simulink model "Simulink_TEP"  (R2024a)
settings: Solver=FixedStepAuto  StartTime=0.0  StopTime=5  FixedStep=1/3600  RelTol=1e-3
model workspace (MAT data in the model file):
  AD : Simulink.Parameter (value not decoded)
  AG : Simulink.Parameter (value not decoded)
  AH : Simulink.Parameter (value not decoded)
  AV : Simulink.Parameter (value not decoded)
  AVP : Simulink.Parameter (value not decoded)
  BCHL : Simulink.Parameter (value not decoded)
  BCHV : Simulink.Parameter (value not decoded)
  BD : Simulink.Parameter (value not decoded)
  BG : Simulink.Parameter (value not decoded)
  BH : Simulink.Parameter (value not decoded)
  BVP : Simulink.Parameter (value not decoded)
  CD : Simulink.Parameter (value not decoded)
  CG : Simulink.Parameter (value not decoded)
  CH : Simulink.Parameter (value not decoded)
  CVP : Simulink.Parameter (value not decoded)
  XMW : Simulink.Parameter (value not decoded)
symbols that are objects in the model workspace (value not decoded): AD, AG, AH, AV, AVP, BD, BG, BH, BVP, CD, CG, CH, CVP, XMW
undefined symbols (not defined in the file or in its folder): magnitude, SETPT, XMEAS, XMV
libraries: mylib x165, dspindex x17
(part 7 of 10)

== system Simulink_TEP/Subsystem/Braatz/ 7 ==
  XMEAS : Inport
  Bus Selector : BusSelector  OutputSignals=signal4.XMEAS(17)
  CONTROL 11 : Subsystem
  XMV(11) : Outport  VectorParamsAs1DForOutWhenUnconnected=off
  wires:
  CONTROL 11/1(XMV(11)) -> XMV(11)/1
  XMEAS/1 -> Bus Selector/1
  Bus Selector/1 -> CONTROL 11/1(XMEAS(17))  "<XMEAS(17)>"

== system Simulink_TEP/Subsystem/Braatz/ 8 ==
  XMEAS : Inport
  Bus Selector : BusSelector  OutputSignals=XMEAS(21),signal2.XMEAS(9)
  CONTROL 10 : Subsystem
  CONTROL 18 : Subsystem
  XMV(10) : Outport  VectorParamsAs1DForOutWhenUnconnected=off
  wires:
  CONTROL 10/1(XMV(10)) -> XMV(10)/1
  CONTROL 18/1(SETPT(10)) -> CONTROL 10/2(SETPT(10))
  XMEAS/1 -> Bus Selector/1
  Bus Selector/1 -> CONTROL 10/1(XMEAS(21))  "<XMEAS(21)>"
  Bus Selector/2 -> CONTROL 18/1(XMEAS(9))  "<XMEAS(9)>"

== system Simulink_TEP/Subsystem/Braatz/ 9 ==
  XMEAS : Inport
  Bus Selector : BusSelector  OutputSignals=signal4.XMEAS(19),signal4.XMEAS(18),signal10.XMEAS(38)
  CONTROL 16 : Subsystem
  CONTROL 20 : Subsystem
  CONTROL 9 : Subsystem
  XMV(9) : Outport  VectorParamsAs1DForOutWhenUnconnected=off
  wires:
  CONTROL 9/1(XMV(9)) -> XMV(9)/1
  CONTROL 16/1(SETPT(9)) -> CONTROL 9/2(SETPT(9))
  XMEAS/1 -> Bus Selector/1
  Bus Selector/1 -> CONTROL 9/1(XMEAS(19))  "<XMEAS(19)>"
  Bus Selector/2 -> CONTROL 16/1(XMEAS(18))  "<XMEAS(18)>"
  Bus Selector/3 -> CONTROL 20/1(XMEAS(38))  "<XMEAS(38)>"
  CONTROL 20/1(SETPT(16)) -> CONTROL 16/2(SETPT(16))

== system Simulink_TEP/Disturbances/Subsystem1/Subsystem2/If Action Subsystem ==
  IDWLK : Inport
  "DIST " : Inport  Port=2
  TESUB7 : Inport  Port=3
  Action Port : ActionPort  ActionPortLabel=elseif(u1 >= u2)
  Bus Creator : BusCreator  Inputs=6
  Bus Selector : BusSelector  OutputSignals=ADIST,BDIST,CDIST,DDIST,TNEXT,TLAST
  Disturbance parameters I=1-9 : mylib/Disturbance parameters I=1-9  SystemSampleTime=-1  VariantActivationTime=update diagram  AllowFlexibleInterface=on  Latency=0  AutoFrameSizeCalculation=off
  Subsystem : Subsystem
      mask Display: color('Blue'),disp('Disturbance constants')
  DIST_NEW : Outport  PortDimensions=6  VectorParamsAs1DForOutWhenUnconnected=off
  wires:
  Disturbance parameters I=1-9/5 -> Bus Creator/5  "TNEXT"
  Bus Creator/1 -> DIST_NEW/1
  IDWLK/1 -> Disturbance parameters I=1-9/7
  Bus Selector/1 -> Disturbance parameters I=1-9/1  "<ADIST>"
  Subsystem/1(Out1) -> Disturbance parameters I=1-9/8
  Bus Selector/2 -> Disturbance parameters I=1-9/2  "<BDIST>"
  Disturbance parameters I=1-9/1 -> Bus Creator/1  "ADIST"
  Bus Selector/6 -> Disturbance parameters I=1-9/6  "<TLAST>"
  Bus Selector/5 -> Disturbance parameters I=1-9/5  "<TNEXT>"
  Disturbance parameters I=1-9/4 -> Bus Creator/4  "DDIST"
  Disturbance parameters I=1-9/3 -> Bus Creator/3  "CDIST"
  Bus Selector/4 -> Disturbance parameters I=1-9/4  "<DDIST>"
  Disturbance parameters I=1-9/6 -> Bus Creator/6  "TLAST"
  Bus Selector/3 -> Disturbance parameters I=1-9/3  "<CDIST>"
  "DIST "/1 -> Bus Selector/1
  Disturbance parameters I=1-9/2 -> Bus Creator/2  "BDIST"
  TESUB7/1 -> Disturbance parameters I=1-9/9

== system Simulink_TEP/Disturbances/Subsystem1/Subsystem2/If Action Subsystem1 ==
  Action Port : ActionPort  ActionPortLabel=if(u1 == 0)
  Subsystem1 : Subsystem
  DIST : Outport  VectorParamsAs1DForOutWhenUnconnected=off
  wires:
  Subsystem1/1(DIST) -> DIST/1

== system Simulink_TEP/Disturbances/Subsystem10/Subsystem3/If Action Subsystem ==
  IDWLK : Inport
  "DIST " : Inport  Port=2
  TESUB7 : Inport  Port=3
  Action Port : ActionPort  ActionPortLabel=elseif(u1 >= u2)
  Bus Creator : BusCreator  Inputs=6
  Bus Selector : BusSelector  OutputSignals=ADIST,BDIST,CDIST,DDIST,TNEXT,TLAST
  Disturbance parameters I=10-12 : mylib/Disturbance parameters I=10-12  SystemSampleTime=-1  VariantActivationTime=update diagram  AllowFlexibleInterface=on  Latency=0  AutoFrameSizeCalculation=off
  Subsystem2 : Subsystem
      mask Display: color('Blue'),disp('Disturbance constants')
  DIST_NEW : Outport  PortDimensions=6  VectorParamsAs1DForOutWhenUnconnected=off
  SWLK : Outport  Port=2  VectorParamsAs1DForOutWhenUnconnected=off
  wires:
  Disturbance parameters I=10-12/5 -> Bus Creator/5  "TNEXT"
  Bus Creator/1 -> DIST_NEW/1
  IDWLK/1 -> Disturbance parameters I=10-12/7
  Bus Selector/1 -> Disturbance parameters I=10-12/1  "<ADIST>"
  Subsystem2/1(Out1) -> Disturbance parameters I=10-12/8
  Bus Selector/2 -> Disturbance parameters I=10-12/2  "<BDIST>"
  Disturbance parameters I=10-12/1 -> Bus Creator/1  "ADIST"
  Bus Selector/6 -> Disturbance parameters I=10-12/6  "<TLAST>"
  Bus Selector/5 -> Disturbance parameters I=10-12/5  "<TNEXT>"
  Disturbance parameters I=10-12/4 -> Bus Creator/4  "DDIST"
  Disturbance parameters I=10-12/3 -> Bus Creator/3  "CDIST"
  Bus Selector/4 -> Disturbance parameters I=10-12/4  "<DDIST>"
  Disturbance parameters I=10-12/6 -> Bus Creator/6  "TLAST"
  Bus Selector/3 -> Disturbance parameters I=10-12/3  "<CDIST>"
  "DIST "/1 -> Bus Selector/1
  Disturbance parameters I=10-12/2 -> Bus Creator/2  "BDIST"
  TESUB7/1 -> Disturbance parameters I=10-12/9
  Disturbance parameters I=10-12/7 -> SWLK/1  "SWLK"

== system Simulink_TEP/Disturbances/Subsystem10/Subsystem3/If Action Subsystem1 ==
  Action Port : ActionPort  ActionPortLabel=if(u1 == 0)
  Subsystem1 : Subsystem
  DIST : Outport  VectorParamsAs1DForOutWhenUnconnected=off
  wires:
  Subsystem1/1(DIST) -> DIST/1

== system Simulink_TEP/Disturbances/Subsystem11/Subsystem3/If Action Subsystem ==
  IDWLK : Inport
  "DIST " : Inport  Port=2
  TESUB7 : Inport  Port=3
  Action Port : ActionPort  ActionPortLabel=elseif(u1 >= u2)
  Bus Creator : BusCreator  Inputs=6
  Bus Selector : BusSelector  OutputSignals=ADIST,BDIST,CDIST,DDIST,TNEXT,TLAST
  Disturbance parameters I=10-12 : mylib/Disturbance parameters I=10-12  SystemSampleTime=-1  VariantActivationTime=update diagram  AllowFlexibleInterface=on  Latency=0  AutoFrameSizeCalculation=off
  Subsystem2 : Subsystem
      mask Display: color('Blue'),disp('Disturbance constants')
  DIST_NEW : Outport  PortDimensions=6  VectorParamsAs1DForOutWhenUnconnected=off
  SWLK : Outport  Port=2  VectorParamsAs1DForOutWhenUnconnected=off
  wires:
  Disturbance parameters I=10-12/5 -> Bus Creator/5  "TNEXT"
  Bus Creator/1 -> DIST_NEW/1
  IDWLK/1 -> Disturbance parameters I=10-12/7
  Bus Selector/1 -> Disturbance parameters I=10-12/1  "<ADIST>"
  Subsystem2/1(Out1) -> Disturbance parameters I=10-12/8
  Bus Selector/2 -> Disturbance parameters I=10-12/2  "<BDIST>"
  Disturbance parameters I=10-12/1 -> Bus Creator/1  "ADIST"
  Bus Selector/6 -> Disturbance parameters I=10-12/6  "<TLAST>"
  Bus Selector/5 -> Disturbance parameters I=10-12/5  "<TNEXT>"
  Disturbance parameters I=10-12/4 -> Bus Creator/4  "DDIST"
  Disturbance parameters I=10-12/3 -> Bus Creator/3  "CDIST"
  Bus Selector/4 -> Disturbance parameters I=10-12/4  "<DDIST>"
  Disturbance parameters I=10-12/6 -> Bus Creator/6  "TLAST"
  Bus Selector/3 -> Disturbance parameters I=10-12/3  "<CDIST>"
  "DIST "/1 -> Bus Selector/1
  Disturbance parameters I=10-12/2 -> Bus Creator/2  "BDIST"
  TESUB7/1 -> Disturbance parameters I=10-12/9
  Disturbance parameters I=10-12/7 -> SWLK/1  "SWLK"

== system Simulink_TEP/Disturbances/Subsystem11/Subsystem3/If Action Subsystem1 ==
  Action Port : ActionPort  ActionPortLabel=if(u1 == 0)
  Subsystem1 : Subsystem
  DIST : Outport  VectorParamsAs1DForOutWhenUnconnected=off
  wires:
  Subsystem1/1(DIST) -> DIST/1

== system Simulink_TEP/Disturbances/Subsystem12/Subsystem3/If Action Subsystem ==
  IDWLK : Inport
  "DIST " : Inport  Port=2
  TESUB7 : Inport  Port=3
  Action Port : ActionPort  ActionPortLabel=elseif(u1 >= u2)
  Bus Creator : BusCreator  Inputs=6
  Bus Selector : BusSelector  OutputSignals=ADIST,BDIST,CDIST,DDIST,TNEXT,TLAST
  Disturbance parameters I=10-12 : mylib/Disturbance parameters I=10-12  SystemSampleTime=-1  VariantActivationTime=update diagram  AllowFlexibleInterface=on  Latency=0  AutoFrameSizeCalculation=off
  Subsystem2 : Subsystem
      mask Display: color('Blue'),disp('Disturbance constants')
  DIST_NEW : Outport  PortDimensions=6  VectorParamsAs1DForOutWhenUnconnected=off
  SWLK : Outport  Port=2  VectorParamsAs1DForOutWhenUnconnected=off
  wires:
  Disturbance parameters I=10-12/5 -> Bus Creator/5  "TNEXT"
  Bus Creator/1 -> DIST_NEW/1
  IDWLK/1 -> Disturbance parameters I=10-12/7
  Bus Selector/1 -> Disturbance parameters I=10-12/1  "<ADIST>"
  Subsystem2/1(Out1) -> Disturbance parameters I=10-12/8
  Bus Selector/2 -> Disturbance parameters I=10-12/2  "<BDIST>"
  Disturbance parameters I=10-12/1 -> Bus Creator/1  "ADIST"
  Bus Selector/6 -> Disturbance parameters I=10-12/6  "<TLAST>"
  Bus Selector/5 -> Disturbance parameters I=10-12/5  "<TNEXT>"
  Disturbance parameters I=10-12/4 -> Bus Creator/4  "DDIST"
  Disturbance parameters I=10-12/3 -> Bus Creator/3  "CDIST"
  Bus Selector/4 -> Disturbance parameters I=10-12/4  "<DDIST>"
  Disturbance parameters I=10-12/6 -> Bus Creator/6  "TLAST"
  Bus Selector/3 -> Disturbance parameters I=10-12/3  "<CDIST>"
  "DIST "/1 -> Bus Selector/1
  Disturbance parameters I=10-12/2 -> Bus Creator/2  "BDIST"
  TESUB7/1 -> Disturbance parameters I=10-12/9
  Disturbance parameters I=10-12/7 -> SWLK/1  "SWLK"

== system Simulink_TEP/Disturbances/Subsystem12/Subsystem3/If Action Subsystem1 ==
  Action Port : ActionPort  ActionPortLabel=if(u1 == 0)
  Subsystem1 : Subsystem
  DIST : Outport  VectorParamsAs1DForOutWhenUnconnected=off
  wires:
  Subsystem1/1(DIST) -> DIST/1

== system Simulink_TEP/Disturbances/Subsystem2/Subsystem/If Action Subsystem ==
  IDWLK : Inport
  "DIST " : Inport  Port=2
  TESUB7 : Inport  Port=3
  Action Port : ActionPort  ActionPortLabel=elseif(u1 >= u2)
  Bus Creator : BusCreator  Inputs=6
  Bus Selector : BusSelector  OutputSignals=ADIST,BDIST,CDIST,DDIST,TNEXT,TLAST
  Disturbance parameters I=1-9 : mylib/Disturbance parameters I=1-9  SystemSampleTime=-1  VariantActivationTime=update diagram  AllowFlexibleInterface=on  Latency=0  AutoFrameSizeCalculation=off
  Subsystem : Subsystem
      mask Display: color('Blue'),disp('Disturbance constants')
  DIST_NEW : Outport  PortDimensions=6  VectorParamsAs1DForOutWhenUnconnected=off
  wires:
  Disturbance parameters I=1-9/5 -> Bus Creator/5  "TNEXT"
  Bus Creator/1 -> DIST_NEW/1
  IDWLK/1 -> Disturbance parameters I=1-9/7
  Bus Selector/1 -> Disturbance parameters I=1-9/1  "<ADIST>"
  Subsystem/1(Out1) -> Disturbance parameters I=1-9/8
  Bus Selector/2 -> Disturbance parameters I=1-9/2  "<BDIST>"
  Disturbance parameters I=1-9/1 -> Bus Creator/1  "ADIST"
  Bus Selector/6 -> Disturbance parameters I=1-9/6  "<TLAST>"
  Bus Selector/5 -> Disturbance parameters I=1-9/5  "<TNEXT>"
  Disturbance parameters I=1-9/4 -> Bus Creator/4  "DDIST"
  Disturbance parameters I=1-9/3 -> Bus Creator/3  "CDIST"
  Bus Selector/4 -> Disturbance parameters I=1-9/4  "<DDIST>"
  Disturbance parameters I=1-9/6 -> Bus Creator/6  "TLAST"
  Bus Selector/3 -> Disturbance parameters I=1-9/3  "<CDIST>"
  "DIST "/1 -> Bus Selector/1
  Disturbance parameters I=1-9/2 -> Bus Creator/2  "BDIST"
  TESUB7/1 -> Disturbance parameters I=1-9/9

== system Simulink_TEP/Disturbances/Subsystem2/Subsystem/If Action Subsystem1 ==
  Action Port : ActionPort  ActionPortLabel=if(u1 == 0)
  Subsystem1 : Subsystem
  DIST : Outport  VectorParamsAs1DForOutWhenUnconnected=off
  wires:
  Subsystem1/1(DIST) -> DIST/1

== system Simulink_TEP/Disturbances/Subsystem3/Subsystem2/If Action Subsystem ==
  IDWLK : Inport
  "DIST " : Inport  Port=2
  TESUB7 : Inport  Port=3
  Action Port : ActionPort  ActionPortLabel=elseif(u1 >= u2)
  Bus Creator : BusCreator  Inputs=6
  Bus Selector : BusSelector  OutputSignals=ADIST,BDIST,CDIST,DDIST,TNEXT,TLAST
  Disturbance parameters I=1-9 : mylib/Disturbance parameters I=1-9  SystemSampleTime=-1  VariantActivationTime=update diagram  AllowFlexibleInterface=on  Latency=0  AutoFrameSizeCalculation=off
  Subsystem : Subsystem
      mask Display: color('Blue'),disp('Disturbance constants')
  DIST_NEW : Outport  PortDimensions=6  VectorParamsAs1DForOutWhenUnconnected=off
  wires:
  Disturbance parameters I=1-9/5 -> Bus Creator/5  "TNEXT"
  Bus Creator/1 -> DIST_NEW/1
  IDWLK/1 -> Disturbance parameters I=1-9/7
  Bus Selector/1 -> Disturbance parameters I=1-9/1  "<ADIST>"
  Subsystem/1(Out1) -> Disturbance parameters I=1-9/8
  Bus Selector/2 -> Disturbance parameters I=1-9/2  "<BDIST>"
  Disturbance parameters I=1-9/1 -> Bus Creator/1  "ADIST"
  Bus Selector/6 -> Disturbance parameters I=1-9/6  "<TLAST>"
  Bus Selector/5 -> Disturbance parameters I=1-9/5  "<TNEXT>"
  Disturbance parameters I=1-9/4 -> Bus Creator/4  "DDIST"
  Disturbance parameters I=1-9/3 -> Bus Creator/3  "CDIST"
  Bus Selector/4 -> Disturbance parameters I=1-9/4  "<DDIST>"
  Disturbance parameters I=1-9/6 -> Bus Creator/6  "TLAST"
  Bus Selector/3 -> Disturbance parameters I=1-9/3  "<CDIST>"
  "DIST "/1 -> Bus Selector/1
  Disturbance parameters I=1-9/2 -> Bus Creator/2  "BDIST"
  TESUB7/1 -> Disturbance parameters I=1-9/9

== system Simulink_TEP/Disturbances/Subsystem3/Subsystem2/If Action Subsystem1 ==
  Action Port : ActionPort  ActionPortLabel=if(u1 == 0)
  Subsystem1 : Subsystem
  DIST : Outport  VectorParamsAs1DForOutWhenUnconnected=off
  wires:
  Subsystem1/1(DIST) -> DIST/1

== system Simulink_TEP/Disturbances/Subsystem4/Subsystem2/If Action Subsystem ==
  IDWLK : Inport
  "DIST " : Inport  Port=2
  TESUB7 : Inport  Port=3
  Action Port : ActionPort  ActionPortLabel=elseif(u1 >= u2)
  Bus Creator : BusCreator  Inputs=6
  Bus Selector : BusSelector  OutputSignals=ADIST,BDIST,CDIST,DDIST,TNEXT,TLAST
  Disturbance parameters I=1-9 : mylib/Disturbance parameters I=1-9  SystemSampleTime=-1  VariantActivationTime=update diagram  AllowFlexibleInterface=on  Latency=0  AutoFrameSizeCalculation=off
  Subsystem : Subsystem
      mask Display: color('Blue'),disp('Disturbance constants')
  DIST_NEW : Outport  PortDimensions=6  VectorParamsAs1DForOutWhenUnconnected=off
  wires:
  Disturbance parameters I=1-9/5 -> Bus Creator/5  "TNEXT"
  Bus Creator/1 -> DIST_NEW/1
  IDWLK/1 -> Disturbance parameters I=1-9/7
  Bus Selector/1 -> Disturbance parameters I=1-9/1  "<ADIST>"
  Subsystem/1(Out1) -> Disturbance parameters I=1-9/8
  Bus Selector/2 -> Disturbance parameters I=1-9/2  "<BDIST>"
  Disturbance parameters I=1-9/1 -> Bus Creator/1  "ADIST"
  Bus Selector/6 -> Disturbance parameters I=1-9/6  "<TLAST>"
  Bus Selector/5 -> Disturbance parameters I=1-9/5  "<TNEXT>"
  Disturbance parameters I=1-9/4 -> Bus Creator/4  "DDIST"
  Disturbance parameters I=1-9/3 -> Bus Creator/3  "CDIST"
  Bus Selector/4 -> Disturbance parameters I=1-9/4  "<DDIST>"
  Disturbance parameters I=1-9/6 -> Bus Creator/6  "TLAST"
  Bus Selector/3 -> Disturbance parameters I=1-9/3  "<CDIST>"
  "DIST "/1 -> Bus Selector/1
  Disturbance parameters I=1-9/2 -> Bus Creator/2  "BDIST"
  TESUB7/1 -> Disturbance parameters I=1-9/9

== system Simulink_TEP/Disturbances/Subsystem4/Subsystem2/If Action Subsystem1 ==
  Action Port : ActionPort  ActionPortLabel=if(u1 == 0)
  Subsystem1 : Subsystem
  DIST : Outport  VectorParamsAs1DForOutWhenUnconnected=off
  wires:
  Subsystem1/1(DIST) -> DIST/1

== system Simulink_TEP/Disturbances/Subsystem5/Subsystem2/If Action Subsystem ==
  IDWLK : Inport
  "DIST " : Inport  Port=2
  TESUB7 : Inport  Port=3
  Action Port : ActionPort  ActionPortLabel=elseif(u1 >= u2)
  Bus Creator : BusCreator  Inputs=6
  Bus Selector : BusSelector  OutputSignals=ADIST,BDIST,CDIST,DDIST,TNEXT,TLAST
  Disturbance parameters I=1-9 : mylib/Disturbance parameters I=1-9  SystemSampleTime=-1  VariantActivationTime=update diagram  AllowFlexibleInterface=on  Latency=0  AutoFrameSizeCalculation=off
  Subsystem : Subsystem
      mask Display: color('Blue'),disp('Disturbance constants')
  DIST_NEW : Outport  PortDimensions=6  VectorParamsAs1DForOutWhenUnconnected=off
  wires:
  Disturbance parameters I=1-9/5 -> Bus Creator/5  "TNEXT"
  Bus Creator/1 -> DIST_NEW/1
  IDWLK/1 -> Disturbance parameters I=1-9/7
  Bus Selector/1 -> Disturbance parameters I=1-9/1  "<ADIST>"
  Subsystem/1(Out1) -> Disturbance parameters I=1-9/8
  Bus Selector/2 -> Disturbance parameters I=1-9/2  "<BDIST>"
  Disturbance parameters I=1-9/1 -> Bus Creator/1  "ADIST"
  Bus Selector/6 -> Disturbance parameters I=1-9/6  "<TLAST>"
  Bus Selector/5 -> Disturbance parameters I=1-9/5  "<TNEXT>"
  Disturbance parameters I=1-9/4 -> Bus Creator/4  "DDIST"
  Disturbance parameters I=1-9/3 -> Bus Creator/3  "CDIST"
  Bus Selector/4 -> Disturbance parameters I=1-9/4  "<DDIST>"
  Disturbance parameters I=1-9/6 -> Bus Creator/6  "TLAST"
  Bus Selector/3 -> Disturbance parameters I=1-9/3  "<CDIST>"
  "DIST "/1 -> Bus Selector/1
  Disturbance parameters I=1-9/2 -> Bus Creator/2  "BDIST"
  TESUB7/1 -> Disturbance parameters I=1-9/9

== system Simulink_TEP/Disturbances/Subsystem5/Subsystem2/If Action Subsystem1 ==
  Action Port : ActionPort  ActionPortLabel=if(u1 == 0)
  Subsystem1 : Subsystem
  DIST : Outport  VectorParamsAs1DForOutWhenUnconnected=off
  wires:
  Subsystem1/1(DIST) -> DIST/1

== system Simulink_TEP/Disturbances/Subsystem6/Subsystem2/If Action Subsystem ==
  IDWLK : Inport
  "DIST " : Inport  Port=2
  TESUB7 : Inport  Port=3
  Action Port : ActionPort  ActionPortLabel=elseif(u1 >= u2)
  Bus Creator : BusCreator  Inputs=6
  Bus Selector : BusSelector  OutputSignals=ADIST,BDIST,CDIST,DDIST,TNEXT,TLAST
  Disturbance parameters I=1-9 : mylib/Disturbance parameters I=1-9  SystemSampleTime=-1  VariantActivationTime=update diagram  AllowFlexibleInterface=on  Latency=0  AutoFrameSizeCalculation=off
  Subsystem : Subsystem
      mask Display: color('Blue'),disp('Disturbance constants')
  DIST_NEW : Outport  PortDimensions=6  VectorParamsAs1DForOutWhenUnconnected=off
  wires:
  Disturbance parameters I=1-9/5 -> Bus Creator/5  "TNEXT"
  Bus Creator/1 -> DIST_NEW/1
  IDWLK/1 -> Disturbance parameters I=1-9/7
  Bus Selector/1 -> Disturbance parameters I=1-9/1  "<ADIST>"
  Subsystem/1(Out1) -> Disturbance parameters I=1-9/8
  Bus Selector/2 -> Disturbance parameters I=1-9/2  "<BDIST>"
  Disturbance parameters I=1-9/1 -> Bus Creator/1  "ADIST"
  Bus Selector/6 -> Disturbance parameters I=1-9/6  "<TLAST>"
  Bus Selector/5 -> Disturbance parameters I=1-9/5  "<TNEXT>"
  Disturbance parameters I=1-9/4 -> Bus Creator/4  "DDIST"
  Disturbance parameters I=1-9/3 -> Bus Creator/3  "CDIST"
  Bus Selector/4 -> Disturbance parameters I=1-9/4  "<DDIST>"
  Disturbance parameters I=1-9/6 -> Bus Creator/6  "TLAST"
  Bus Selector/3 -> Disturbance parameters I=1-9/3  "<CDIST>"
  "DIST "/1 -> Bus Selector/1
  Disturbance parameters I=1-9/2 -> Bus Creator/2  "BDIST"
  TESUB7/1 -> Disturbance parameters I=1-9/9

== system Simulink_TEP/Disturbances/Subsystem6/Subsystem2/If Action Subsystem1 ==
  Action Port : ActionPort  ActionPortLabel=if(u1 == 0)
  Subsystem1 : Subsystem
  DIST : Outport  VectorParamsAs1DForOutWhenUnconnected=off
  wires:
  Subsystem1/1(DIST) -> DIST/1

== system Simulink_TEP/Disturbances/Subsystem7/Subsystem2/If Action Subsystem ==
  IDWLK : Inport
  "DIST " : Inport  Port=2
  TESUB7 : Inport  Port=3
  Action Port : ActionPort  ActionPortLabel=elseif(u1 >= u2)
  Bus Creator : BusCreator  Inputs=6
  Bus Selector : BusSelector  OutputSignals=ADIST,BDIST,CDIST,DDIST,TNEXT,TLAST
  Disturbance parameters I=1-9 : mylib/Disturbance parameters I=1-9  SystemSampleTime=-1  VariantActivationTime=update diagram  AllowFlexibleInterface=on  Latency=0  AutoFrameSizeCalculation=off
  Subsystem : Subsystem
      mask Display: color('Blue'),disp('Disturbance constants')
  DIST_NEW : Outport  PortDimensions=6  VectorParamsAs1DForOutWhenUnconnected=off
  wires:
  Disturbance parameters I=1-9/5 -> Bus Creator/5  "TNEXT"
  Bus Creator/1 -> DIST_NEW/1
  IDWLK/1 -> Disturbance parameters I=1-9/7
  Bus Selector/1 -> Disturbance parameters I=1-9/1  "<ADIST>"
  Subsystem/1(Out1) -> Disturbance parameters I=1-9/8
  Bus Selector/2 -> Disturbance parameters I=1-9/2  "<BDIST>"
  Disturbance parameters I=1-9/1 -> Bus Creator/1  "ADIST"
  Bus Selector/6 -> Disturbance parameters I=1-9/6  "<TLAST>"
  Bus Selector/5 -> Disturbance parameters I=1-9/5  "<TNEXT>"
  Disturbance parameters I=1-9/4 -> Bus Creator/4  "DDIST"
  Disturbance parameters I=1-9/3 -> Bus Creator/3  "CDIST"
  Bus Selector/4 -> Disturbance parameters I=1-9/4  "<DDIST>"
  Disturbance parameters I=1-9/6 -> Bus Creator/6  "TLAST"
  Bus Selector/3 -> Disturbance parameters I=1-9/3  "<CDIST>"
  "DIST "/1 -> Bus Selector/1
  Disturbance parameters I=1-9/2 -> Bus Creator/2  "BDIST"
  TESUB7/1 -> Disturbance parameters I=1-9/9

== system Simulink_TEP/Disturbances/Subsystem7/Subsystem2/If Action Subsystem1 ==
  Action Port : ActionPort  ActionPortLabel=if(u1 == 0)
  Subsystem1 : Subsystem
  DIST : Outport  VectorParamsAs1DForOutWhenUnconnected=off
  wires:
  Subsystem1/1(DIST) -> DIST/1

== system Simulink_TEP/Disturbances/Subsystem8/Subsystem2/If Action Subsystem ==
  IDWLK : Inport
  "DIST " : Inport  Port=2
  TESUB7 : Inport  Port=3
  Action Port : ActionPort  ActionPortLabel=elseif(u1 >= u2)
  Bus Creator : BusCreator  Inputs=6
  Bus Selector : BusSelector  OutputSignals=ADIST,BDIST,CDIST,DDIST,TNEXT,TLAST
  Disturbance parameters I=1-9 : mylib/Disturbance parameters I=1-9  SystemSampleTime=-1  VariantActivationTime=update diagram  AllowFlexibleInterface=on  Latency=0  AutoFrameSizeCalculation=off
  Subsystem : Subsystem
      mask Display: color('Blue'),disp('Disturbance constants')
  DIST_NEW : Outport  PortDimensions=6  VectorParamsAs1DForOutWhenUnconnected=off
  wires:
  Disturbance parameters I=1-9/5 -> Bus Creator/5  "TNEXT"
  Bus Creator/1 -> DIST_NEW/1
  IDWLK/1 -> Disturbance parameters I=1-9/7
  Bus Selector/1 -> Disturbance parameters I=1-9/1  "<ADIST>"
  Subsystem/1(Out1) -> Disturbance parameters I=1-9/8
  Bus Selector/2 -> Disturbance parameters I=1-9/2  "<BDIST>"
  Disturbance parameters I=1-9/1 -> Bus Creator/1  "ADIST"
  Bus Selector/6 -> Disturbance parameters I=1-9/6  "<TLAST>"
  Bus Selector/5 -> Disturbance parameters I=1-9/5  "<TNEXT>"
  Disturbance parameters I=1-9/4 -> Bus Creator/4  "DDIST"
  Disturbance parameters I=1-9/3 -> Bus Creator/3  "CDIST"
  Bus Selector/4 -> Disturbance parameters I=1-9/4  "<DDIST>"
  Disturbance parameters I=1-9/6 -> Bus Creator/6  "TLAST"
  Bus Selector/3 -> Disturbance parameters I=1-9/3  "<CDIST>"
  "DIST "/1 -> Bus Selector/1
  Disturbance parameters I=1-9/2 -> Bus Creator/2  "BDIST"
  TESUB7/1 -> Disturbance parameters I=1-9/9

== system Simulink_TEP/Disturbances/Subsystem8/Subsystem2/If Action Subsystem1 ==
  Action Port : ActionPort  ActionPortLabel=if(u1 == 0)
  Subsystem1 : Subsystem
  DIST : Outport  VectorParamsAs1DForOutWhenUnconnected=off
  wires:
  Subsystem1/1(DIST) -> DIST/1

== system Simulink_TEP/Disturbances/Subsystem9/Subsystem2/If Action Subsystem ==
  IDWLK : Inport
  "DIST " : Inport  Port=2
  TESUB7 : Inport  Port=3
  Action Port : ActionPort  ActionPortLabel=elseif(u1 >= u2)
  Bus Creator : BusCreator  Inputs=6
  Bus Selector : BusSelector  OutputSignals=ADIST,BDIST,CDIST,DDIST,TNEXT,TLAST
  Disturbance parameters I=1-9 : mylib/Disturbance parameters I=1-9  SystemSampleTime=-1  VariantActivationTime=update diagram  AllowFlexibleInterface=on  Latency=0  AutoFrameSizeCalculation=off
  Subsystem : Subsystem
      mask Display: color('Blue'),disp('Disturbance constants')
  DIST_NEW : Outport  PortDimensions=6  VectorParamsAs1DForOutWhenUnconnected=off
  wires:
  Disturbance parameters I=1-9/5 -> Bus Creator/5  "TNEXT"
  Bus Creator/1 -> DIST_NEW/1
  IDWLK/1 -> Disturbance parameters I=1-9/7
  Bus Selector/1 -> Disturbance parameters I=1-9/1  "<ADIST>"
  Subsystem/1(Out1) -> Disturbance parameters I=1-9/8
  Bus Selector/2 -> Disturbance parameters I=1-9/2  "<BDIST>"
  Disturbance parameters I=1-9/1 -> Bus Creator/1  "ADIST"
  Bus Selector/6 -> Disturbance parameters I=1-9/6  "<TLAST>"
  Bus Selector/5 -> Disturbance parameters I=1-9/5  "<TNEXT>"
  Disturbance parameters I=1-9/4 -> Bus Creator/4  "DDIST"
  Disturbance parameters I=1-9/3 -> Bus Creator/3  "CDIST"
  Bus Selector/4 -> Disturbance parameters I=1-9/4  "<DDIST>"
  Disturbance parameters I=1-9/6 -> Bus Creator/6  "TLAST"
  Bus Selector/3 -> Disturbance parameters I=1-9/3  "<CDIST>"
  "DIST "/1 -> Bus Selector/1
  Disturbance parameters I=1-9/2 -> Bus Creator/2  "BDIST"
  TESUB7/1 -> Disturbance parameters I=1-9/9

== system Simulink_TEP/Disturbances/Subsystem9/Subsystem2/If Action Subsystem1 ==
  Action Port : ActionPort  ActionPortLabel=if(u1 == 0)
  Subsystem1 : Subsystem
  DIST : Outport  VectorParamsAs1DForOutWhenUnconnected=off
  wires:
  Subsystem1/1(DIST) -> DIST/1

== system Simulink_TEP/Mixing Zone/Stream 6/Subsystem/If Action Subsystem ==
  In1 : Inport
  Action Port : ActionPort  ActionPortLabel=if(u1 < 0)
  Out1 : Outport  VectorParamsAs1DForOutWhenUnconnected=off
  wires:
  In1/1 -> Out1/1

== system Simulink_TEP/Mixing Zone/Stream 6/Subsystem/If Action Subsystem1 ==
  In1 : Inport
  Action Port : ActionPort  ActionPortLabel=else
  Out1 : Outport  VectorParamsAs1DForOutWhenUnconnected=off
  wires:
  In1/1 -> Out1/1

== system Simulink_TEP/Process Measurements/Feed Streams/D Feed/XMWS(1) Molecular weight of Stream 1 lb//lb-mol ==
  XST(I,1) : Inport
  Product : Product
  Sum of Elements : Sum  Inputs=+
  "XMW(I) Molecular weight of components lb/lb-mol " : Constant  Value=XMW
  XMWS(1) : Outport  VectorParamsAs1DForOutWhenUnconnected=off
  wires:
  Sum of Elements/1 -> XMWS(1)/1
  Product/1 -> Sum of Elements/1
  XST(I,1)/1 -> Product/1
  "XMW(I) Molecular weight of components lb/lb-mol "/1 -> Product/2

== system Simulink_TEP/Process Measurements/Feed Streams/E Feed/XMWS(2) Molecular weight of Stream 2 lb//lb-mol ==
  XST(I,2) : Inport
  Product : Product
  Sum of Elements : Sum  Inputs=+
  "XMW(I) Molecular weight of components lb/lb-mol " : Constant  Value=XMW
  XMWS(2) : Outport  VectorParamsAs1DForOutWhenUnconnected=off
  wires:
  Sum of Elements/1 -> XMWS(2)/1
  Product/1 -> Sum of Elements/1
  XST(I,2)/1 -> Product/1
  "XMW(I) Molecular weight of components lb/lb-mol "/1 -> Product/2

== system Simulink_TEP/Process Measurements/Product analysis/Subsystem/Subsystem ==
  XST : Inport
  Constant : Constant  Value=100
  Multiport Selector : dspindex/Multiport Selector  rowsOrCols=Rows  idxCellArray={4,5,6,7,8}  idxErrMode=Clip Index
  XCMP(37) : Product
  XCMP(38) : Product
  XCMP(39) : Product
  XCMP(40) : Product
  XCMP(41) : Product
  "XCMP(37) " : Outport  VectorParamsAs1DForOutWhenUnconnected=off
  "XCMP(38) " : Outport  Port=2  VectorParamsAs1DForOutWhenUnconnected=off
  "XCMP(39) " : Outport  Port=3  VectorParamsAs1DForOutWhenUnconnected=off
  "XCMP(40) " : Outport  Port=4  VectorParamsAs1DForOutWhenUnconnected=off
  "XCMP(41) " : Outport  Port=5  VectorParamsAs1DForOutWhenUnconnected=off
  wires:
  Constant/1 -> XCMP(38)/2, XCMP(40)/2, XCMP(41)/2, XCMP(39)/2, XCMP(37)/2
  Multiport Selector/1 -> XCMP(37)/1
  XCMP(37)/1 -> "XCMP(37) "/1  "XCMP(37)"
  Multiport Selector/5 -> XCMP(41)/1
  XCMP(39)/1 -> "XCMP(39) "/1  "XCMP(39)"
  XST/1 -> Multiport Selector/1
  Multiport Selector/4 -> XCMP(40)/1
  Multiport Selector/2 -> XCMP(38)/1
  Multiport Selector/3 -> XCMP(39)/1
  XCMP(38)/1 -> "XCMP(38) "/1  "XCMP(38)"
  XCMP(41)/1 -> "XCMP(41) "/1  "XCMP(41)"
  XCMP(40)/1 -> "XCMP(40) "/1  "XCMP(40)"

== system Simulink_TEP/Process Measurements/Purge gas analysis/Subsystem/Subsystem ==
  XST : Inport
  Constant : Constant  Value=100
  Multiport Selector : dspindex/Multiport Selector  rowsOrCols=Rows  idxCellArray={ 1,2,3,4,5,6,7,8}  idxErrMode=Clip Index
  XCMP(29) : Product
  XCMP(30) : Product
  XCMP(31) : Product
  XCMP(32) : Product
  XCMP(33) : Product
  XCMP(34) : Product
  XCMP(35) : Product
  XCMP(36) : Product
  "XCMP(29) " : Outport  VectorParamsAs1DForOutWhenUnconnected=off
  "XCMP(30) " : Outport  Port=2  VectorParamsAs1DForOutWhenUnconnected=off
  "XCMP(31) " : Outport  Port=3  VectorParamsAs1DForOutWhenUnconnected=off
  "XCMP(32) " : Outport  Port=4  VectorParamsAs1DForOutWhenUnconnected=off
  "XCMP(33) " : Outport  Port=5  VectorParamsAs1DForOutWhenUnconnected=off
  "XCMP(34) " : Outport  Port=6  VectorParamsAs1DForOutWhenUnconnected=off
  "XCMP(35) " : Outport  Port=7  VectorParamsAs1DForOutWhenUnconnected=off
  "XCMP(36) " : Outport  Port=8  VectorParamsAs1DForOutWhenUnconnected=off
  wires:
  XCMP(32)/1 -> "XCMP(32) "/1  "XCMP(32)"
  Multiport Selector/6 -> XCMP(34)/1
  Multiport Selector/8 -> XCMP(36)/1
  XCMP(29)/1 -> "XCMP(29) "/1  "XCMP(29)"
  Multiport Selector/5 -> XCMP(33)/1
  Multiport Selector/7 -> XCMP(35)/1
  XCMP(30)/1 -> "XCMP(30) "/1  "XCMP(30)"
  Multiport Selector/1 -> XCMP(29)/1
  Multiport Selector/3 -> XCMP(31)/1
  Constant/1 -> XCMP(32)/2, XCMP(36)/2, XCMP(35)/2, XCMP(34)/2, XCMP(33)/2, XCMP(31)/2, XCMP(30)/2, XCMP(29)/2
  XCMP(33)/1 -> "XCMP(33) "/1  "XCMP(33)"
  Multiport Selector/4 -> XCMP(32)/1
  XST/1 -> Multiport Selector/1
  Multiport Selector/2 -> XCMP(30)/1
  XCMP(31)/1 -> "XCMP(31) "/1  "XCMP(31)"
  XCMP(35)/1 -> "XCMP(35) "/1  "XCMP(35)"
  XCMP(36)/1 -> "XCMP(36) "/1  "XCMP(36)"
  XCMP(34)/1 -> "XCMP(34) "/1  "XCMP(34)"

== system Simulink_TEP/Process Measurements/Reactor feed analysis/Subsystem/Subsystem ==
  XST : Inport
  Constant : Constant  Value=100
  Multiport Selector : dspindex/Multiport Selector  rowsOrCols=Rows  idxCellArray={ 1,2,3,4,5,6,}  idxErrMode=Clip Index
  XCMP(23) : Product
  XCMP(24) : Product
  XCMP(25) : Product
  XCMP(26) : Product
  XCMP(27) : Product
  XCMP(28) : Product
  XCMP(23)1 : Outport  VectorParamsAs1DForOutWhenUnconnected=off
  XCMP(24)1 : Outport  Port=2  VectorParamsAs1DForOutWhenUnconnected=off
  XCMP(25)1 : Outport  Port=3  VectorParamsAs1DForOutWhenUnconnected=off
  XCMP(26)1 : Outport  Port=4  VectorParamsAs1DForOutWhenUnconnected=off
  XCMP(27)1 : Outport  Port=5  VectorParamsAs1DForOutWhenUnconnected=off
  XCMP(28)1 : Outport  Port=6  VectorParamsAs1DForOutWhenUnconnected=off
  wires:
  Multiport Selector/1 -> XCMP(23)/1  "XST(1;7)"
  Multiport Selector/4 -> XCMP(26)/1  "XST(4;7)"
  Constant/1 -> XCMP(26)/2, XCMP(28)/2, XCMP(27)/2, XCMP(25)/2, XCMP(24)/2, XCMP(23)/2
  Multiport Selector/2 -> XCMP(24)/1  "XST(2;7)"
  XST/1 -> Multiport Selector/1
  Multiport Selector/6 -> XCMP(28)/1  "XST(6:7)"
  Multiport Selector/3 -> XCMP(25)/1  "XST(3;7)"
  XCMP(23)/1 -> XCMP(23)1/1  "XCMP(23)"
  Multiport Selector/5 -> XCMP(27)/1  "XST(5;7)"
  XCMP(25)/1 -> XCMP(25)1/1  "XCMP(25)"
  XCMP(26)/1 -> XCMP(26)1/1  "XCMP(26)"
  XCMP(24)/1 -> XCMP(24)1/1  "XCMP(24)"
  XCMP(27)/1 -> XCMP(27)1/1  "XCMP(27)"
  XCMP(28)/1 -> XCMP(28)1/1  "XCMP(28)"

== system Simulink_TEP/Random number generator/Disturbances I=1-9/TESUB7(1)/If Action Subsystem3 ==
  G : Inport
  Action Port : ActionPort  ActionPortLabel=if(u1 ~= 0 & u1 >= u2)
  Constant : Constant  Value=-1
  TESUB7 G-New : mylib/TESUB7 G-New  SystemSampleTime=-1  VariantActivationTime=update diagram  AllowFlexibleInterface=on  Latency=0  AutoFrameSizeCalculation=off
  TESUB7(1) : Outport  VectorParamsAs1DForOutWhenUnconnected=off
  G_NEW : Outport  Port=2  OutputWhenDisabled=reset  InitialOutput=[0]  VectorParamsAs1DForOutWhenUnconnected=off
  wires:
  Constant/1 -> TESUB7 G-New/1
  G/1 -> TESUB7 G-New/2
  TESUB7 G-New/2 -> G_NEW/1
  TESUB7 G-New/1 -> TESUB7(1)/1

== system Simulink_TEP/Random number generator/Disturbances I=1-9/TESUB7(1)/Subsystem ==
  In2 : Inport
  G : Inport  Port=2
  If Action Subsystem : Subsystem  TreatAsAtomicUnit=on
  If Action Subsystem1 : Subsystem  TreatAsAtomicUnit=on
  If5 : If  IfExpression=u1 == 0
  Merge : Merge
  G1 : Outport  VectorParamsAs1DForOutWhenUnconnected=off
  wires:
  In2/1 -> If Action Subsystem1/1(In1), If5/1
  If5/2 -> If Action Subsystem1/Action
  If Action Subsystem1/1(Out1) -> Merge/1
  If5/1 -> If Action Subsystem/Action
  If Action Subsystem/1(Out1) -> Merge/2
  G/1 -> If Action Subsystem/1(In1)
  Merge/1 -> G1/1

== system Simulink_TEP/Random number generator/Disturbances I=1-9/TESUB7(1)/TNEXT(1) ==
  Bus Selector : BusSelector  OutputSignals=TNEXT
  Clock3 : Clock
  If3 : If  NumInputs=2  IfExpression=u1 ~= 0 & u1 >= u2  ShowElse=off
  IF(1) : Outport  VectorParamsAs1DForOutWhenUnconnected=off
  wires:
  Bus Selector/1 -> If3/2  "<TNEXT>"
  Clock3/1 -> If3/1
  If3/1 -> IF(1)/1
  [DIST1] -> Bus Selector/1

== system Simulink_TEP/Random number generator/Disturbances I=1-9/TESUB7(2)/If Action Subsystem3 ==
  G : Inport
  Action Port : ActionPort  ActionPortLabel=if(u1 ~= 0 & u1 >= u2)
  Constant : Constant  Value=-1
  TESUB7 G-New : mylib/TESUB7 G-New  SystemSampleTime=-1  VariantActivationTime=update diagram  AllowFlexibleInterface=on  Latency=0  AutoFrameSizeCalculation=off
  TESUB7(2) : Outport  VectorParamsAs1DForOutWhenUnconnected=off
  G_NEW : Outport  Port=2  OutputWhenDisabled=reset  InitialOutput=[0]  VectorParamsAs1DForOutWhenUnconnected=off
  wires:
  Constant/1 -> TESUB7 G-New/1
  G/1 -> TESUB7 G-New/2
  TESUB7 G-New/2 -> G_NEW/1
  TESUB7 G-New/1 -> TESUB7(2)/1

== system Simulink_TEP/Random number generator/Disturbances I=1-9/TESUB7(2)/Subsystem ==
  In2 : Inport
  G : Inport  Port=2
  If Action Subsystem : Subsystem  TreatAsAtomicUnit=on
  If Action Subsystem1 : Subsystem  TreatAsAtomicUnit=on
  If5 : If  IfExpression=u1 == 0
  Merge : Merge
  G1 : Outport  VectorParamsAs1DForOutWhenUnconnected=off
  wires:
  In2/1 -> If Action Subsystem1/1(In1), If5/1
  If5/2 -> If Action Subsystem1/Action
  If Action Subsystem1/1(Out1) -> Merge/1
  If5/1 -> If Action Subsystem/Action
  If Action Subsystem/1(Out1) -> Merge/2
  G/1 -> If Action Subsystem/1(In1)
  Merge/1 -> G1/1

== system Simulink_TEP/Random number generator/Disturbances I=1-9/TESUB7(2)/TNEXT(2) ==
  Bus Selector : BusSelector  OutputSignals=TNEXT
  Clock3 : Clock
  If3 : If  NumInputs=2  IfExpression=u1 ~= 0 & u1 >= u2  ShowElse=off
  IF(2) : Outport  VectorParamsAs1DForOutWhenUnconnected=off
  wires:
  Bus Selector/1 -> If3/2  "<TNEXT>"
  Clock3/1 -> If3/1
  If3/1 -> IF(2)/1
  [DIST2] -> Bus Selector/1

== system Simulink_TEP/Random number generator/Disturbances I=1-9/TESUB7(3)/If Action Subsystem3 ==
  G : Inport
  Action Port : ActionPort  ActionPortLabel=if(u1 ~= 0 & u1 >= u2)
  Constant : Constant  Value=-1
  TESUB7 G-New : mylib/TESUB7 G-New  SystemSampleTime=-1  VariantActivationTime=update diagram  AllowFlexibleInterface=on  Latency=0  AutoFrameSizeCalculation=off
  TESUB7(3) : Outport  VectorParamsAs1DForOutWhenUnconnected=off
  G_NEW : Outport  Port=2  OutputWhenDisabled=reset  InitialOutput=[0]  VectorParamsAs1DForOutWhenUnconnected=off
  wires:
  Constant/1 -> TESUB7 G-New/1
  G/1 -> TESUB7 G-New/2
  TESUB7 G-New/2 -> G_NEW/1
  TESUB7 G-New/1 -> TESUB7(3)/1

== system Simulink_TEP/Random number generator/Disturbances I=1-9/TESUB7(3)/Subsystem ==
  In2 : Inport
  G : Inport  Port=2
  If Action Subsystem : Subsystem  TreatAsAtomicUnit=on
  If Action Subsystem1 : Subsystem  TreatAsAtomicUnit=on
  If5 : If  IfExpression=u1 == 0
  Merge : Merge
  G1 : Outport  VectorParamsAs1DForOutWhenUnconnected=off
  wires:
  In2/1 -> If Action Subsystem1/1(In1), If5/1
  If5/2 -> If Action Subsystem1/Action
  If Action Subsystem1/1(Out1) -> Merge/1
  If5/1 -> If Action Subsystem/Action
  If Action Subsystem/1(Out1) -> Merge/2
  G/1 -> If Action Subsystem/1(In1)
  Merge/1 -> G1/1

== system Simulink_TEP/Random number generator/Disturbances I=1-9/TESUB7(3)/TNEXT(3) ==
  Bus Selector : BusSelector  OutputSignals=TNEXT
  Clock3 : Clock
  If3 : If  NumInputs=2  IfExpression=u1 ~= 0 & u1 >= u2  ShowElse=off
  IF(3) : Outport  VectorParamsAs1DForOutWhenUnconnected=off
  wires:
  Bus Selector/1 -> If3/2  "<TNEXT>"
  Clock3/1 -> If3/1
  If3/1 -> IF(3)/1
  [DIST3] -> Bus Selector/1

== system Simulink_TEP/Random number generator/Disturbances I=1-9/TESUB7(4)/If Action Subsystem3 ==
  G : Inport
  Action Port : ActionPort  ActionPortLabel=if(u1 ~= 0 & u1 >= u2)
  Constant : Constant  Value=-1
  TESUB7 G-New : mylib/TESUB7 G-New  SystemSampleTime=-1  VariantActivationTime=update diagram  AllowFlexibleInterface=on  Latency=0  AutoFrameSizeCalculation=off
  TESUB7(4) : Outport  VectorParamsAs1DForOutWhenUnconnected=off
  G_NEW : Outport  Port=2  OutputWhenDisabled=reset  InitialOutput=[0]  VectorParamsAs1DForOutWhenUnconnected=off
  wires:
  Constant/1 -> TESUB7 G-New/1
  G/1 -> TESUB7 G-New/2
  TESUB7 G-New/2 -> G_NEW/1
  TESUB7 G-New/1 -> TESUB7(4)/1

== system Simulink_TEP/Random number generator/Disturbances I=1-9/TESUB7(4)/Subsystem ==
  In2 : Inport
  G : Inport  Port=2
  If Action Subsystem : Subsystem  TreatAsAtomicUnit=on
  If Action Subsystem1 : Subsystem  TreatAsAtomicUnit=on
  If5 : If  IfExpression=u1 == 0
  Merge : Merge
  G1 : Outport  VectorParamsAs1DForOutWhenUnconnected=off
  wires:
  In2/1 -> If Action Subsystem1/1(In1), If5/1
  If5/2 -> If Action Subsystem1/Action
  If Action Subsystem1/1(Out1) -> Merge/1
  If5/1 -> If Action Subsystem/Action
  If Action Subsystem/1(Out1) -> Merge/2
  G/1 -> If Action Subsystem/1(In1)
  Merge/1 -> G1/1

== system Simulink_TEP/Random number generator/Disturbances I=1-9/TESUB7(4)/TNEXT(4) ==
  Bus Selector : BusSelector  OutputSignals=TNEXT
  Clock3 : Clock
  If3 : If  NumInputs=2  IfExpression=u1 ~= 0 & u1 >= u2  ShowElse=off
  IF(4) : Outport  VectorParamsAs1DForOutWhenUnconnected=off
  wires:
  Bus Selector/1 -> If3/2  "<TNEXT>"
  Clock3/1 -> If3/1
  If3/1 -> IF(4)/1
  [DIST4] -> Bus Selector/1

== system Simulink_TEP/Random number generator/Disturbances I=1-9/TESUB7(5)/If Action Subsystem3 ==
  G : Inport
  Action Port : ActionPort  ActionPortLabel=if(u1 ~= 0 & u1 >= u2)
  Constant : Constant  Value=-1
  TESUB7 G-New : mylib/TESUB7 G-New  SystemSampleTime=-1  VariantActivationTime=update diagram  AllowFlexibleInterface=on  Latency=0  AutoFrameSizeCalculation=off
  TESUB7(5) : Outport  VectorParamsAs1DForOutWhenUnconnected=off
  G_NEW : Outport  Port=2  OutputWhenDisabled=reset  InitialOutput=[0]  VectorParamsAs1DForOutWhenUnconnected=off
  wires:
  Constant/1 -> TESUB7 G-New/1
  G/1 -> TESUB7 G-New/2
  TESUB7 G-New/2 -> G_NEW/1
  TESUB7 G-New/1 -> TESUB7(5)/1

== system Simulink_TEP/Random number generator/Disturbances I=1-9/TESUB7(5)/Subsystem ==
  In2 : Inport
  G : Inport  Port=2
  If Action Subsystem : Subsystem  TreatAsAtomicUnit=on
  If Action Subsystem1 : Subsystem  TreatAsAtomicUnit=on
  If5 : If  IfExpression=u1 == 0
  Merge : Merge
  G1 : Outport  VectorParamsAs1DForOutWhenUnconnected=off
  wires:
  In2/1 -> If Action Subsystem1/1(In1), If5/1
  If5/2 -> If Action Subsystem1/Action
  If Action Subsystem1/1(Out1) -> Merge/1
  If5/1 -> If Action Subsystem/Action
  If Action Subsystem/1(Out1) -> Merge/2
  G/1 -> If Action Subsystem/1(In1)
  Merge/1 -> G1/1

== system Simulink_TEP/Random number generator/Disturbances I=1-9/TESUB7(5)/TNEXT(5) ==
  Bus Selector : BusSelector  OutputSignals=TNEXT
  Clock3 : Clock
  If3 : If  NumInputs=2  IfExpression=u1 ~= 0 & u1 >= u2  ShowElse=off
  IF(5) : Outport  VectorParamsAs1DForOutWhenUnconnected=off
  wires:
  Bus Selector/1 -> If3/2  "<TNEXT>"
  Clock3/1 -> If3/1
  If3/1 -> IF(5)/1
  [DIST5] -> Bus Selector/1

== system Simulink_TEP/Random number generator/Disturbances I=1-9/TESUB7(6)/If Action Subsystem3 ==
  G : Inport
  Action Port : ActionPort  ActionPortLabel=if(u1 ~= 0 & u1 >= u2)
  Constant : Constant  Value=-1
  TESUB7 G-New : mylib/TESUB7 G-New  SystemSampleTime=-1  VariantActivationTime=update diagram  AllowFlexibleInterface=on  Latency=0  AutoFrameSizeCalculation=off
  TESUB7(6) : Outport  VectorParamsAs1DForOutWhenUnconnected=off
  G_NEW : Outport  Port=2  OutputWhenDisabled=reset  InitialOutput=[0]  VectorParamsAs1DForOutWhenUnconnected=off
  wires:
  Constant/1 -> TESUB7 G-New/1
  G/1 -> TESUB7 G-New/2
  TESUB7 G-New/2 -> G_NEW/1
  TESUB7 G-New/1 -> TESUB7(6)/1

== system Simulink_TEP/Random number generator/Disturbances I=1-9/TESUB7(6)/Subsystem ==
  In2 : Inport
  G : Inport  Port=2
  If Action Subsystem : Subsystem  TreatAsAtomicUnit=on
  If Action Subsystem1 : Subsystem  TreatAsAtomicUnit=on
  If5 : If  IfExpression=u1 == 0
  Merge : Merge
  G1 : Outport  VectorParamsAs1DForOutWhenUnconnected=off
  wires:
  In2/1 -> If Action Subsystem1/1(In1), If5/1
  If5/2 -> If Action Subsystem1/Action
  If Action Subsystem1/1(Out1) -> Merge/1
  If5/1 -> If Action Subsystem/Action
  If Action Subsystem/1(Out1) -> Merge/2
  G/1 -> If Action Subsystem/1(In1)
  Merge/1 -> G1/1

== system Simulink_TEP/Random number generator/Disturbances I=1-9/TESUB7(6)/TNEXT(6) ==
  Bus Selector : BusSelector  OutputSignals=TNEXT
  Clock3 : Clock
  If3 : If  NumInputs=2  IfExpression=u1 ~= 0 & u1 >= u2  ShowElse=off
  IF(6) : Outport  VectorParamsAs1DForOutWhenUnconnected=off
  wires:
  Bus Selector/1 -> If3/2  "<TNEXT>"
  Clock3/1 -> If3/1
  If3/1 -> IF(6)/1
  [DIST6] -> Bus Selector/1

== system Simulink_TEP/Random number generator/Disturbances I=1-9/TESUB7(7)/If Action Subsystem3 ==
  G : Inport
  Action Port : ActionPort  ActionPortLabel=if(u1 ~= 0 & u1 >= u2)
  Constant : Constant  Value=-1
  TESUB7 G-New : mylib/TESUB7 G-New  SystemSampleTime=-1  VariantActivationTime=update diagram  AllowFlexibleInterface=on  Latency=0  AutoFrameSizeCalculation=off
  TESUB7(7) : Outport  VectorParamsAs1DForOutWhenUnconnected=off
  G_NEW : Outport  Port=2  OutputWhenDisabled=reset  InitialOutput=[0]  VectorParamsAs1DForOutWhenUnconnected=off
  wires:
  Constant/1 -> TESUB7 G-New/1
  G/1 -> TESUB7 G-New/2
  TESUB7 G-New/2 -> G_NEW/1
  TESUB7 G-New/1 -> TESUB7(7)/1

== system Simulink_TEP/Random number generator/Disturbances I=1-9/TESUB7(7)/Subsystem ==
  In2 : Inport
  G : Inport  Port=2
  If Action Subsystem : Subsystem  TreatAsAtomicUnit=on
  If Action Subsystem1 : Subsystem  TreatAsAtomicUnit=on
  If5 : If  IfExpression=u1 == 0
  Merge : Merge
  G1 : Outport  VectorParamsAs1DForOutWhenUnconnected=off
  wires:
  In2/1 -> If Action Subsystem1/1(In1), If5/1
  If5/2 -> If Action Subsystem1/Action
  If Action Subsystem1/1(Out1) -> Merge/1
  If5/1 -> If Action Subsystem/Action
  If Action Subsystem/1(Out1) -> Merge/2
  G/1 -> If Action Subsystem/1(In1)
  Merge/1 -> G1/1

== system Simulink_TEP/Random number generator/Disturbances I=1-9/TESUB7(7)/TNEXT(7) ==
  Bus Selector : BusSelector  OutputSignals=TNEXT
  Clock3 : Clock
  If3 : If  NumInputs=2  IfExpression=u1 ~= 0 & u1 >= u2  ShowElse=off
  IF(7) : Outport  VectorParamsAs1DForOutWhenUnconnected=off
  wires:
  Bus Selector/1 -> If3/2  "<TNEXT>"
  Clock3/1 -> If3/1
  If3/1 -> IF(7)/1
  [DIST7] -> Bus Selector/1

== system Simulink_TEP/Random number generator/Disturbances I=1-9/TESUB7(8)/If Action Subsystem3 ==
  G : Inport
  Action Port : ActionPort  ActionPortLabel=if(u1 ~= 0 & u1 >= u2)
  Constant : Constant  Value=-1
  TESUB7 G-New : mylib/TESUB7 G-New  SystemSampleTime=-1  VariantActivationTime=update diagram  AllowFlexibleInterface=on  Latency=0  AutoFrameSizeCalculation=off
  TESUB7(8) : Outport  VectorParamsAs1DForOutWhenUnconnected=off
  G_NEW : Outport  Port=2  OutputWhenDisabled=reset  InitialOutput=[0]  VectorParamsAs1DForOutWhenUnconnected=off
  wires:
  Constant/1 -> TESUB7 G-New/1
  G/1 -> TESUB7 G-New/2
  TESUB7 G-New/2 -> G_NEW/1
  TESUB7 G-New/1 -> TESUB7(8)/1

== system Simulink_TEP/Random number generator/Disturbances I=1-9/TESUB7(8)/Subsystem ==
  In2 : Inport
  G : Inport  Port=2
  If Action Subsystem : Subsystem  TreatAsAtomicUnit=on
  If Action Subsystem1 : Subsystem  TreatAsAtomicUnit=on
  If5 : If  IfExpression=u1 == 0
  Merge : Merge
  G1 : Outport  VectorParamsAs1DForOutWhenUnconnected=off
  wires:
  In2/1 -> If Action Subsystem1/1(In1), If5/1
  If5/2 -> If Action Subsystem1/Action
  If Action Subsystem1/1(Out1) -> Merge/1
  If5/1 -> If Action Subsystem/Action
  If Action Subsystem/1(Out1) -> Merge/2
  G/1 -> If Action Subsystem/1(In1)
  Merge/1 -> G1/1

== system Simulink_TEP/Random number generator/Disturbances I=1-9/TESUB7(8)/TNEXT(8) ==
  Bus Selector : BusSelector  OutputSignals=TNEXT
  Clock3 : Clock
  If3 : If  NumInputs=2  IfExpression=u1 ~= 0 & u1 >= u2  ShowElse=off
  IF(8) : Outport  VectorParamsAs1DForOutWhenUnconnected=off
  wires:
  Bus Selector/1 -> If3/2  "<TNEXT>"
  Clock3/1 -> If3/1
  If3/1 -> IF(8)/1
  [DIST8] -> Bus Selector/1

== system Simulink_TEP/Random number generator/Disturbances I=1-9/TESUB7(9)/If Action Subsystem3 ==
  G : Inport
  Action Port : ActionPort  ActionPortLabel=if(u1 ~= 0 & u1 >= u2)
  Constant : Constant  Value=-1
  TESUB7 G-New : mylib/TESUB7 G-New  SystemSampleTime=-1  VariantActivationTime=update diagram  AllowFlexibleInterface=on  Latency=0  AutoFrameSizeCalculation=off
  TESUB7(9) : Outport  VectorParamsAs1DForOutWhenUnconnected=off
  G_NEW : Outport  Port=2  OutputWhenDisabled=reset  InitialOutput=[0]  VectorParamsAs1DForOutWhenUnconnected=off
  wires:
  Constant/1 -> TESUB7 G-New/1
  G/1 -> TESUB7 G-New/2
  TESUB7 G-New/2 -> G_NEW/1
  TESUB7 G-New/1 -> TESUB7(9)/1

== system Simulink_TEP/Random number generator/Disturbances I=1-9/TESUB7(9)/Subsystem ==
  In2 : Inport
  G : Inport  Port=2
  If Action Subsystem : Subsystem  TreatAsAtomicUnit=on
  If Action Subsystem1 : Subsystem  TreatAsAtomicUnit=on
  If5 : If  IfExpression=u1 == 0
  Merge : Merge
  G1 : Outport  VectorParamsAs1DForOutWhenUnconnected=off
  wires:
  In2/1 -> If Action Subsystem1/1(In1), If5/1
  If5/2 -> If Action Subsystem1/Action
  If Action Subsystem1/1(Out1) -> Merge/1
  If5/1 -> If Action Subsystem/Action
  If Action Subsystem/1(Out1) -> Merge/2
  G/1 -> If Action Subsystem/1(In1)
  Merge/1 -> G1/1

== system Simulink_TEP/Random number generator/Disturbances I=1-9/TESUB7(9)/TNEXT(9) ==
  Bus Selector : BusSelector  OutputSignals=TNEXT
  Clock3 : Clock
  If3 : If  NumInputs=2  IfExpression=u1 ~= 0 & u1 >= u2  ShowElse=off
  IF(9) : Outport  VectorParamsAs1DForOutWhenUnconnected=off
  wires:
  Bus Selector/1 -> If3/2  "<TNEXT>"
  Clock3/1 -> If3/1
  If3/1 -> IF(9)/1
  [DIST9] -> Bus Selector/1

== system Simulink_TEP/Random number generator/Disturbances I=10-12/TESUB7(10)/If Action Subsystem3 ==
  G : Inport
  Action Port : ActionPort  ActionPortLabel=if(u1 ~= 0 & u1 >= u2 & u3 < 0.1)
  Constant : Constant  Value=-1
  TESUB7 G-New : mylib/TESUB7 G-New  SystemSampleTime=-1  VariantActivationTime=update diagram  AllowFlexibleInterface=on  Latency=0  AutoFrameSizeCalculation=off
  TESUB7(10) : Outport  VectorParamsAs1DForOutWhenUnconnected=off
  G_NEW : Outport  Port=2  OutputWhenDisabled=reset  InitialOutput=[0]  VectorParamsAs1DForOutWhenUnconnected=off
  wires:
  Constant/1 -> TESUB7 G-New/1
  G/1 -> TESUB7 G-New/2
  TESUB7 G-New/2 -> G_NEW/1
  TESUB7 G-New/1 -> TESUB7(10)/1

== system Simulink_TEP/Random number generator/Disturbances I=10-12/TESUB7(10)/Subsystem ==
  In2 : Inport
  G : Inport  Port=2
  If Action Subsystem : Subsystem  TreatAsAtomicUnit=on
  If Action Subsystem1 : Subsystem  TreatAsAtomicUnit=on
  If5 : If  IfExpression=u1 == 0
  Merge : Merge
  G1 : Outport  VectorParamsAs1DForOutWhenUnconnected=off
  wires:
  In2/1 -> If Action Subsystem1/1(In1), If5/1
  If5/2 -> If Action Subsystem1/Action
  If Action Subsystem1/1(Out1) -> Merge/1
  If5/1 -> If Action Subsystem/Action
  If Action Subsystem/1(Out1) -> Merge/2
  G/1 -> If Action Subsystem/1(In1)
  Merge/1 -> G1/1

== system Simulink_TEP/Random number generator/Disturbances I=10-12/TESUB7(10)/TNEXT(10) ==
  Bus Selector : BusSelector  OutputSignals=TNEXT
  Clock3 : Clock
  If3 : If  NumInputs=3  IfExpression=u1 ~= 0 & u1 >= u2 & u3 < 0.1  ShowElse=off
  IF(10) : Outport  VectorParamsAs1DForOutWhenUnconnected=off
  wires:
  Bus Selector/1 -> If3/2  "<TNEXT>"
  Clock3/1 -> If3/1
  If3/1 -> IF(10)/1
  [DIST10] -> Bus Selector/1
  [SWLK_10] -> If3/3

== system Simulink_TEP/Random number generator/Disturbances I=10-12/TESUB7(11)/If Action Subsystem3 ==
  G : Inport
  Action Port : ActionPort  ActionPortLabel=if(u1 ~= 0 & u1 >= u2 & u3 < 0.1)
  Constant : Constant  Value=-1
  TESUB7 G-New : mylib/TESUB7 G-New  SystemSampleTime=-1  VariantActivationTime=update diagram  AllowFlexibleInterface=on  Latency=0  AutoFrameSizeCalculation=off
  TESUB7(11) : Outport  VectorParamsAs1DForOutWhenUnconnected=off
  G_NEW : Outport  Port=2  OutputWhenDisabled=reset  InitialOutput=[0]  VectorParamsAs1DForOutWhenUnconnected=off
  wires:
  Constant/1 -> TESUB7 G-New/1
  G/1 -> TESUB7 G-New/2
  TESUB7 G-New/2 -> G_NEW/1
  TESUB7 G-New/1 -> TESUB7(11)/1
